simulink model "model"  (R2021b)
settings: Solver=VariableStepAuto  StartTime=0.0  StopTime=30  RelTol=1e-3
undefined symbols (not defined in the file): h, mian, ym
settings Model: Creator=szczy  LastModifiedBy=szczy

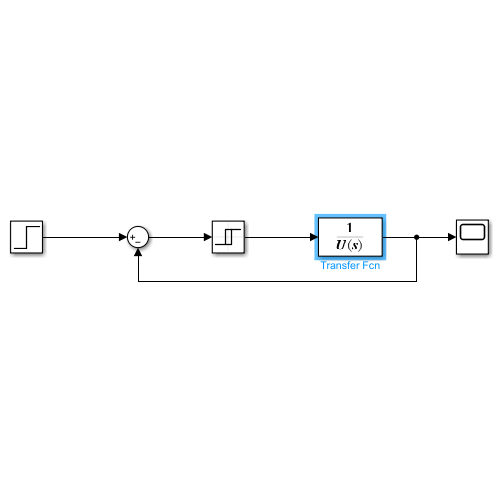
[thumbnail: Simulink's stored preview of the top-level diagram]
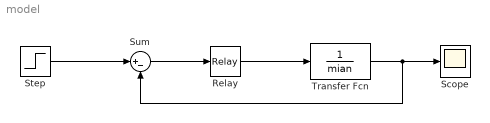
== system model ==
  Relay : Relay  OnSwitchValue=h  OffSwitchValue=-h  OnOutputValue=ym  OffOutputValue=-ym
  Scope : Scope
  Step : Step  SampleTime=0
  Sum : Sum  Inputs=|+-
  Transfer Fcn : TransferFcn  Denominator=mian
  wires:
  Step/1 -> Sum/1
  Sum/1 -> Relay/1
  Relay/1 -> Transfer Fcn/1
  Transfer Fcn/1 -> Sum/2, Scope/1
